simulink model "sampleModel1843"  (R2023a)
settings: Solver=VariableStepAuto  StartTime=0.0  StopTime=10.0  RelTol=1e-3
libraries: hdlsllib x6, simulink x3
settings Model: Creator=user1  LastModifiedBy=user1

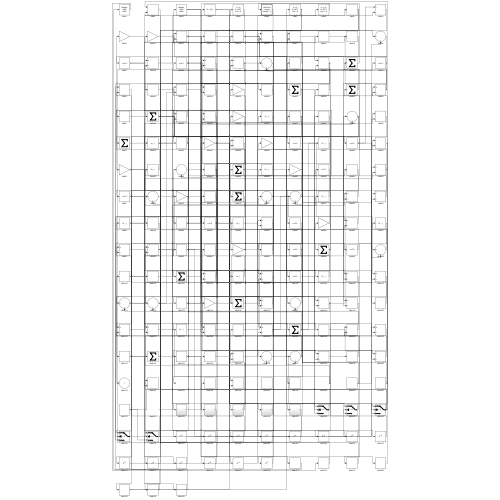
[thumbnail: Simulink's stored preview of the top-level diagram]
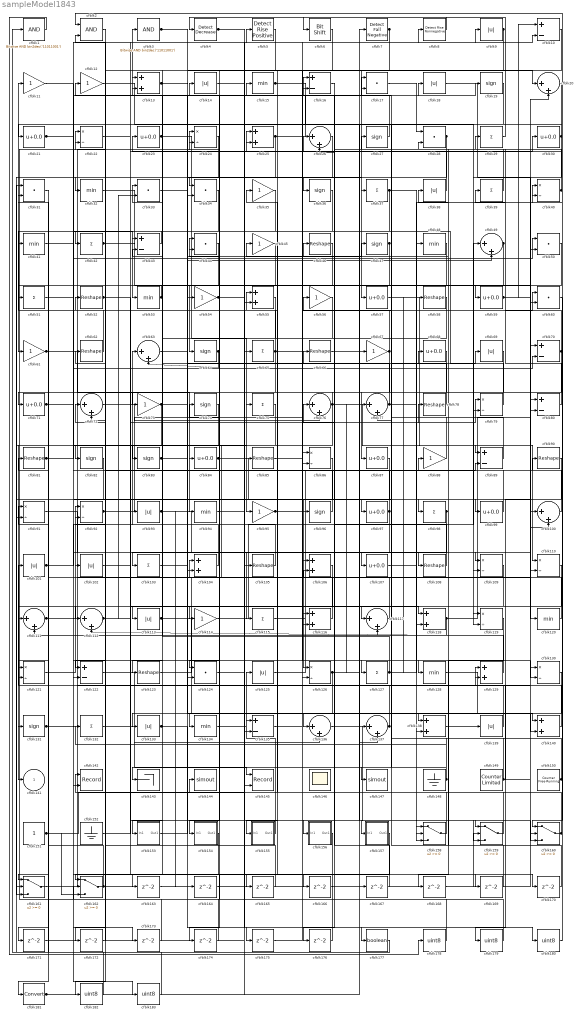
== system sampleModel1843 ==
  cfblk1 : simulink/Logic and Bit Operations/Bitwise Operator  logicop=AND  UseBitMask=on  BitMask=bin2dec('11011001')  BitMaskRealWorld=Stored Integer
      settings: LibrarySourceBlock=|
      | hdlsllib/Logic and Bit
      | Operations/Bitwise
      | Operator
  cfblk{10,16,43,70,80,89,122,135} (8 alike) : Sum  Inputs=+-
  cfblk{20,26,49,63,72,76..77,100,111..112,117,136..137} (13 alike) : Sum  Inputs=|++
  cfblk{9,14,18,38,69,93,101..102,113,125,133,139} (12 alike) : Abs  SaturateOnIntegerOverflow=off
  cfblk{29,37,39,42,51,65,75,98,103,115,127,132} (12 alike) : Sum  Inputs=+
  cfblk{13,25,55,104,106,116,118,129,138,140} (10 alike) : Sum
  cfblk{46,52,58,62,66,78,81,85,90,105,108,123} (12 alike) : Reshape
  cfblk{21,23,30,57,59,68,71,84,87,97,99,107} (12 alike) : Bias  Bias=0.0  SaturateOnIntegerOverflow=off
  cfblk{22,24,40,79,86,91..92,109..110,119,121,126,130} (13 alike) : Product  Inputs=*/  RndMeth=Zero  SaturateOnIntegerOverflow=on
  cfblk{11..12,35,45,54,56,61,67,73,88,95,114} (12 alike) : Gain
  cfblk{15,32,41,48,53,94,120,128,134} (9 alike) : MinMax
  cfblk{17,28,31,33..34,44,50,60,124} (9 alike) : DotProduct  OutDataTypeStr=Inherit: Inherit via internal rule
  cfblk{19,27,36,47,64,74,82..83,96,131} (10 alike) : Signum
  cfblk142 : Record  FileSettingsInternal="{\"entries\":[{\"content\":{\"excelSettings\":{\"content\":{},\"type\":\"Streamout.ExcelSettings\"}},\"type\":\"Streamout.FileSettingStorage\",\"uuid\":\"\"}],\"packageUris\":[\"http:\\/\\/schema.mathworks.com\\/mf0\\/streamout_blocks\\/R2020a\"],\"version\":\"1.0\"}"  Layout=[1 1]  SignalsInternal="{\"entries\":[{\"content\":{\"signals\":[{\"content\":{\"blockPath\":[],\"dimensions\":[1],\"domain\":\"\",\"lineColor\":\"#a2142f\",\"plots\":[1],\"port\":1,\"signalID\":4494,\"signalName\":\"XY Graph:1\"},\"type\":\"RecordBlkView.Signal\",\"uuid\":\"\"},{\"content\":{\"blockPath\":[],\"dimensions\":[1],\"domain\":\"\",\"lineColor\":\"#139fff\",\"plots\":[1],\"port\":2,\"signalID\":4497,\"signalName\":\"XY Graph:2\"},\"type\":\"RecordBlkView.Signal\",\"uuid\":\"\"}]},\"type\":\"RecordBlkView.InputSignals\",\"uuid\":\"\"}],\"packageUris\":[\"http:\\/\\/schema.mathworks.com\\/mf0\\/streamout_blocks\\/R2020a\"],\"version\":\"1.0\"}"  VisualizationBindings="{\"xyplotplugin\":{\"info\":[{\"series\":[{\"bindingParametersList\":[{\"parameter\":\"X-Axis\",\"signalID\":4494,\"signalName\":\"XY Graph:1\"},{\"parameter\":\"Y-Axis\",\"signalID\":4497,\"signalName\":\"XY Graph:2\"}],\"seriesID\":46456}],\"subplotID\":1}]}}"  CompatibilityTag=XY  st=-1
  cfblk143 : Terminator
  cfblk144 : ToWorkspace  VariableName=simout  SaveFormat=Timeseries  SampleTime=-1
  cfblk145 : Record  FileSettingsInternal="{\"entries\":[{\"content\":{\"excelSettings\":{\"content\":{},\"type\":\"Streamout.ExcelSettings\"}},\"type\":\"Streamout.FileSettingStorage\",\"uuid\":\"\"}],\"packageUris\":[\"http:\\/\\/schema.mathworks.com\\/mf0\\/streamout_blocks\\/R2020a\"],\"version\":\"1.0\"}"  Layout=[1 1]  SignalsInternal="{\"entries\":[{\"content\":{\"signals\":[{\"content\":{\"blockPath\":[],\"dimensions\":[1],\"domain\":\"\",\"lineColor\":\"#a2142f\",\"plots\":[1],\"port\":1,\"signalID\":4502,\"signalName\":\"XY Graph:1\"},\"type\":\"RecordBlkView.Signal\",\"uuid\":\"\"},{\"content\":{\"blockPath\":[],\"dimensions\":[1],\"domain\":\"\",\"lineColor\":\"#139fff\",\"plots\":[1],\"port\":2,\"signalID\":4505,\"signalName\":\"XY Graph:2\"},\"type\":\"RecordBlkView.Signal\",\"uuid\":\"\"}]},\"type\":\"RecordBlkView.InputSignals\",\"uuid\":\"\"}],\"packageUris\":[\"http:\\/\\/schema.mathworks.com\\/mf0\\/streamout_blocks\\/R2020a\"],\"version\":\"1.0\"}"  VisualizationBindings="{\"xyplotplugin\":{\"info\":[{\"series\":[{\"bindingParametersList\":[{\"parameter\":\"X-Axis\",\"signalID\":4502,\"signalName\":\"XY Graph:1\"},{\"parameter\":\"Y-Axis\",\"signalID\":4505,\"signalName\":\"XY Graph:2\"}],\"seriesID\":46147}],\"subplotID\":1}]}}"  CompatibilityTag=XY  st=-1
  cfblk146 : Scope
      settings: Floating=on
  cfblk147 : ToWorkspace  VariableName=simout  SaveFormat=Timeseries  SampleTime=-1
  cfblk148 : Ground
  cfblk149 : hdlsllib/Sources/Counter Limited  uplimit=7  tsamp=-1
  cfblk150 : hdlsllib/Sources/Counter Free-Running  NumBits=16  tsamp=-1
  cfblk151 : Constant  SampleTime=-1
  cfblk152 : Ground
  cfblk153 : Subsystem
      settings: LibrarySourceBlock=|
      | hdlsllib/Ports &
      | Subsystems/Subsystem
  cfblk154 : Subsystem
      settings: LibrarySourceBlock=|
      | hdlsllib/Ports &
      | Subsystems/Subsystem
  cfblk155 : Subsystem
      settings: LibrarySourceBlock=|
      | hdlsllib/Ports &
      | Subsystems/Subsystem
  cfblk156 : Subsystem
      settings: LibrarySourceBlock=|
      | hdlsllib/Ports &
      | Subsystems/Subsystem
  cfblk157 : Subsystem
      settings: LibrarySourceBlock=|
      | hdlsllib/Ports &
      | Subsystems/Subsystem
  cfblk{158..162} (5 alike) : Switch  SaturateOnIntegerOverflow=off  InputSameDT=off
  cfblk{163..176} (14 alike) : Delay  SampleTime=1
  cfblk177 : DataTypeConversion  OutDataTypeStr=boolean  SaturateOnIntegerOverflow=off  RndMeth=Floor
  cfblk{178..180,182..183} (5 alike) : DataTypeConversion  OutDataTypeStr=uint8  SaturateOnIntegerOverflow=off  RndMeth=Floor
  cfblk181 : DataTypeConversion  SaturateOnIntegerOverflow=off  RndMeth=Floor
  cfblk2 : Logic  AllPortsSameDT=off  OutDataTypeStr=boolean
  cfblk3 : simulink/Logic and Bit Operations/Bitwise Operator  logicop=AND  UseBitMask=on  BitMask=bin2dec('11011001')  BitMaskRealWorld=Stored Integer
      settings: LibrarySourceBlock=|
      | hdlsllib/Logic and Bit
      | Operations/Bitwise
      | Operator
  cfblk4 : simulink/Logic and Bit Operations/Detect Decrease  vinit=0.0  OutDataTypeStr=boolean
      settings: LibrarySourceBlock=|
      | hdlsllib/Logic and Bit
      | Operations/Detect
      | Decrease
  cfblk5 : hdlsllib/Logic and Bit Operations/Detect Rise Positive  vinit=0  OutDataTypeStr=boolean
  cfblk6 : hdlsllib/Logic and Bit Operations/Bit Shift  mode=Shift Left Logical  N=0
  cfblk7 : hdlsllib/Logic and Bit Operations/Detect Fall Negative  vinit=0  OutDataTypeStr=boolean
  cfblk8 : hdlsllib/Logic and Bit Operations/Detect Rise Nonnegative  vinit=0  OutDataTypeStr=boolean
  cfblk141 : Outport  VectorParamsAs1DForOutWhenUnconnected=off
  wires:
  cfblk122/1 -> cfblk145/1
  cfblk161/1 -> cfblk24/1
  cfblk125/1 -> cfblk88/1
  cfblk100/1 -> cfblk45/1
  cfblk126/1 -> cfblk158/3, cfblk77/1, cfblk163/1
  cfblk79/1 -> cfblk53/1
  cfblk9/1 -> cfblk57/1, cfblk116/2
  cfblk99/1 -> cfblk66/1
  cfblk25/1 -> cfblk18/1, cfblk124/1
  cfblk27/1 -> cfblk3/1
  cfblk80/1 -> cfblk39/1
  cfblk47/1 -> cfblk64/1, cfblk122/2
  cfblk58/1 -> cfblk103/1
  cfblk75/1 -> cfblk104/1
  cfblk88/1 -> cfblk23/1
  cfblk57/1 -> cfblk110/1
  cfblk43/1 -> cfblk42/1
  cfblk77/1 -> cfblk52/1, cfblk160/3
  cfblk51/1 -> cfblk50/1
  cfblk130/1 -> cfblk136/1
  cfblk23/1 -> cfblk95/1, cfblk118/1
  cfblk40/1 -> cfblk15/1, cfblk25/2
  cfblk156/1(Out1) -> cfblk22/1
  cfblk46/1 -> cfblk155/1(In1)
  cfblk14/1 -> cfblk107/1
  cfblk31/1 -> cfblk181/1
  cfblk18/1 -> cfblk100/1
  cfblk7/1 -> cfblk34/1, cfblk182/1
  cfblk155/1(Out1) -> cfblk125/1
  cfblk65/1 -> cfblk60/1, cfblk121/1, cfblk43/2
  cfblk72/1 -> cfblk76/2
  cfblk104/1 -> cfblk63/1
  cfblk73/1 -> cfblk141/1, cfblk116/1
  cfblk64/1 -> cfblk63/2, cfblk134/1
  cfblk38/1 -> cfblk25/1
  cfblk103/1 -> cfblk54/1
  cfblk56/1 -> cfblk123/1
  cfblk84/1 -> cfblk120/1, cfblk10/2
  cfblk159/1 -> cfblk55/1
  cfblk52/1 -> cfblk19/1, cfblk160/2
  cfblk24/1 -> cfblk104/2
  cfblk136/1 -> cfblk159/1
  cfblk86/1 -> cfblk126/1
  cfblk93/1 -> cfblk145/2, cfblk140/2, cfblk164/1
  cfblk138/1 -> cfblk139/1
  cfblk128/1 -> cfblk140/1
  cfblk26/1 -> cfblk82/1
  cfblk120/1 -> cfblk44/1
  cfblk110/1 -> cfblk131/1
  cfblk123/1 -> cfblk67/1
  cfblk29/1 -> cfblk4/1
  cfblk55/1 -> cfblk154/1(In1)
  cfblk12/1 -> cfblk137/1
  cfblk137/1 -> cfblk101/1, cfblk16/2
  cfblk121/1 -> cfblk92/1
  cfblk70/1 -> cfblk29/1, cfblk87/1
  cfblk5/1 -> cfblk73/1
  cfblk95/1 -> cfblk35/1, cfblk69/1
  cfblk150/1 -> cfblk2/1, cfblk117/2
  cfblk158/1 -> cfblk44/2
  cfblk116/1 -> cfblk14/1
  cfblk134/1 -> cfblk135/1
  cfblk61/1 -> cfblk94/1, cfblk173/1
  cfblk49/1 -> cfblk96/1, cfblk109/2
  cfblk160/1 -> cfblk142/1, cfblk40/2, cfblk62/1
  cfblk133/1 -> cfblk175/1, cfblk177/1
  cfblk132/1 -> cfblk136/2
  cfblk62/1 -> cfblk11/1
  cfblk148/1 -> cfblk17/1, cfblk132/1, cfblk143/1
  cfblk108/1 -> cfblk26/1
  cfblk37/1 -> cfblk113/1, cfblk99/1
  cfblk92/1 -> cfblk8/1, cfblk118/2
  cfblk44/1 -> cfblk142/2
  cfblk17/1 -> cfblk28/1
  cfblk139/1 -> cfblk91/1
  cfblk81/1 -> cfblk5/1, cfblk89/2
  cfblk45/1 -> cfblk122/1
  cfblk63/1 -> cfblk138/1
  cfblk34/1 -> cfblk61/1
  cfblk91/1 -> cfblk106/1
  cfblk48/1 -> cfblk147/1
  cfblk68/1 -> cfblk117/1
  cfblk2/1 -> cfblk32/1
  cfblk35/1 -> cfblk41/1
  cfblk39/1 -> cfblk12/1
  cfblk69/1 -> cfblk111/1
  cfblk15/1 -> cfblk137/2, cfblk119/1
  cfblk66/1 -> cfblk110/2
  cfblk22/1 -> cfblk9/1
  cfblk87/1 -> cfblk161/1
  cfblk105/1 -> cfblk74/1
  cfblk109/1 -> cfblk153/1(In1)
  cfblk151/1 -> cfblk135/2, cfblk162/3
  cfblk124/1 -> cfblk79/1
  cfblk107/1 -> cfblk158/1
  cfblk82/1 -> cfblk161/2
  cfblk4/1 -> cfblk157/1(In1), cfblk180/1
  cfblk8/1 -> cfblk6/1
  cfblk41/1 -> cfblk85/1
  cfblk89/1 -> cfblk16/1
  cfblk153/1(Out1) -> cfblk47/1
  cfblk162/1 -> cfblk7/1, cfblk121/2
  cfblk10/1 -> cfblk75/1
  cfblk20/1 -> cfblk34/2
  cfblk19/1 -> cfblk97/1
  cfblk102/1 -> cfblk30/1
  cfblk11/1 -> cfblk98/1
  cfblk135/1 -> cfblk129/1
  cfblk114/1 -> cfblk49/1
  cfblk112/1 -> cfblk33/2, cfblk169/1
  cfblk28/1 -> cfblk91/2, cfblk112/1
  cfblk42/1 -> cfblk60/2, cfblk105/1, cfblk119/2
  cfblk152/1 -> cfblk78/1
  cfblk118/1 -> cfblk50/2, cfblk112/2
  cfblk131/1 -> cfblk80/1, cfblk183/1
  cfblk111/1 -> cfblk48/1, cfblk170/1
  cfblk113/1 -> cfblk138/2, cfblk68/1
  cfblk115/1 -> cfblk70/1
  cfblk101/1 -> cfblk93/1, cfblk108/1
  cfblk33/1 -> cfblk128/1
  cfblk36/1 -> cfblk114/1
  cfblk30/1 -> cfblk79/2, cfblk21/1
  cfblk154/1(Out1) -> cfblk162/1
  cfblk67/1 -> cfblk84/1, cfblk26/2
  cfblk32/1 -> cfblk86/2
  cfblk71/1 -> cfblk127/1, cfblk70/2
  cfblk3/1 -> cfblk37/1, cfblk20/1, cfblk109/1
  cfblk60/1 -> cfblk160/1
  cfblk13/1 -> cfblk59/1, cfblk36/1
  cfblk117/1 -> cfblk81/1
  cfblk21/1 -> cfblk13/1, cfblk43/1
  cfblk59/1 -> cfblk100/2, cfblk10/1
  cfblk96/1 -> cfblk24/2
  cfblk94/1 -> cfblk156/1(In1)
  cfblk53/1 -> cfblk83/1, cfblk51/1
  cfblk149/1 -> cfblk56/1, cfblk129/2, cfblk20/2
  cfblk78/1 -> cfblk27/1
  cfblk127/1 -> cfblk40/1, cfblk58/1, cfblk33/1
  cfblk97/1 -> cfblk72/2, cfblk115/1, cfblk176/1
  cfblk54/1 -> cfblk159/3, cfblk158/2
  cfblk85/1 -> cfblk130/2
  cfblk129/1 -> cfblk111/2
  cfblk74/1 -> cfblk161/3
  cfblk98/1 -> cfblk38/1, cfblk124/2
  cfblk140/1 -> cfblk106/2
  cfblk83/1 -> cfblk17/2, cfblk49/2, cfblk13/2
  cfblk76/1 -> cfblk46/1, cfblk89/1, cfblk71/1, cfblk133/1
  cfblk163/1 -> cfblk86/1
  cfblk164/1 -> cfblk80/2
  cfblk106/1 -> cfblk165/1
  cfblk165/1 -> cfblk22/2
  cfblk16/1 -> cfblk166/1
  cfblk166/1 -> cfblk130/1
  cfblk167/1 -> cfblk76/1
  cfblk119/1 -> cfblk168/1
  cfblk168/1 -> cfblk159/2
  cfblk169/1 -> cfblk28/2
  cfblk170/1 -> cfblk77/2
  cfblk50/1 -> cfblk171/1
  cfblk171/1 -> cfblk55/2
  cfblk6/1 -> cfblk172/1
  cfblk172/1 -> cfblk92/2
  cfblk173/1 -> cfblk162/2
  cfblk157/1(Out1) -> cfblk174/1
  cfblk174/1 -> cfblk72/1
  cfblk175/1 -> cfblk126/2
  cfblk176/1 -> cfblk2/2
  cfblk177/1 -> cfblk1/1
  cfblk1/1 -> cfblk178/1
  cfblk178/1 -> cfblk144/1
  cfblk90/1 -> cfblk179/1
  cfblk179/1 -> cfblk102/1
  cfblk180/1 -> cfblk90/1
  cfblk181/1 -> cfblk167/1, cfblk65/1
  cfblk182/1 -> cfblk31/1
  cfblk183/1 -> cfblk31/2

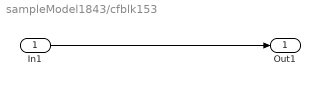
== system sampleModel1843/cfblk153 ==
  In1 : Inport
  Out1 : Outport
  wires:
  In1/1 -> Out1/1

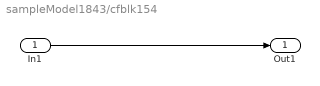
== system sampleModel1843/cfblk154 ==
  In1 : Inport
  Out1 : Outport
  wires:
  In1/1 -> Out1/1

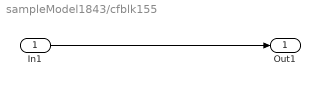
== system sampleModel1843/cfblk155 ==
  In1 : Inport
  Out1 : Outport
  wires:
  In1/1 -> Out1/1

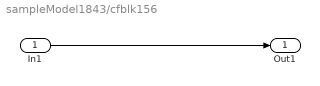
== system sampleModel1843/cfblk156 ==
  In1 : Inport
  Out1 : Outport
  wires:
  In1/1 -> Out1/1

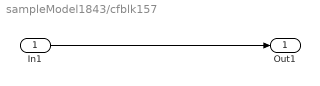
== system sampleModel1843/cfblk157 ==
  In1 : Inport
  Out1 : Outport
  wires:
  In1/1 -> Out1/1
